simulink model "Thandra_Rushika_prelab5"  (R2022a)
settings: Solver=VariableStepAuto  StartTime=0.0  StopTime=1  RelTol=1e-3
libraries: commanapbnd3 x2
settings Model: Creator=rishika  LastModifiedBy=rishika

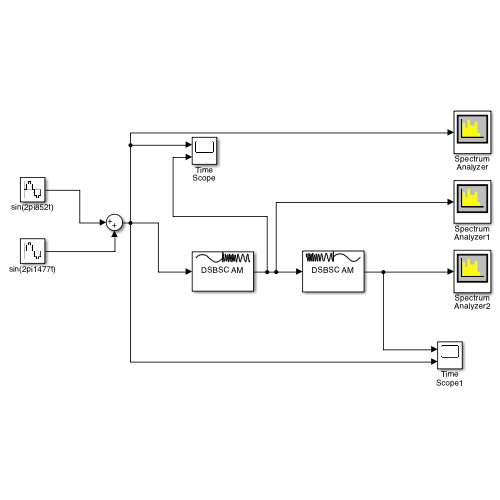
[thumbnail: Simulink's stored preview of the top-level diagram]
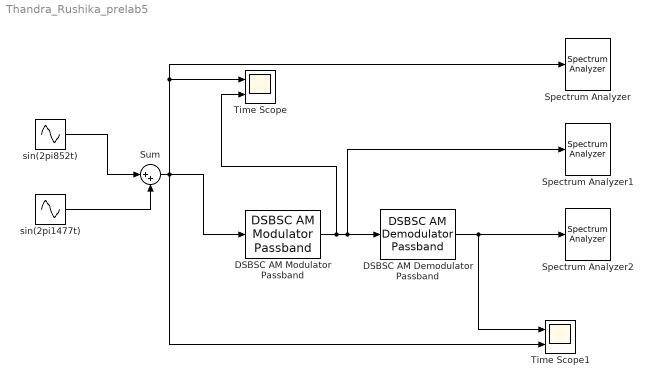
== system Thandra_Rushika_prelab5 ==
  DSBSC AM Demodulator Passband : commanapbnd3/DSBSC AM Demodulator Passband  Fc=8000  Ph=0  method=Butterworth  n=4  cf=5000  Rp=0.1  Rs=50
      settings: SourceProductBaseCode=CM
  DSBSC AM Modulator Passband : commanapbnd3/DSBSC AM Modulator Passband  Fc=8000  Ph=0
      settings: SourceProductBaseCode=CM
  Spectrum Analyzer : SpectrumAnalyzer
  Spectrum Analyzer1 : SpectrumAnalyzer
  Spectrum Analyzer2 : SpectrumAnalyzer
  Sum : Sum  Inputs=|++
  Time Scope : Scope  NumInputPorts=2
  Time Scope1 : Scope  NumInputPorts=2
  sin(2pi1477t) : Sin  Frequency=2*pi*1477  Phase=0.00001  SampleTime=0.00001
  sin(2pi852t) : Sin  Frequency=2*pi*852  SampleTime=0.00001
  wires:
  DSBSC AM Demodulator Passband/1 -> Time Scope1/1, Spectrum Analyzer2/1
  sin(2pi1477t)/1 -> Sum/2
  sin(2pi852t)/1 -> Sum/1
  Sum/1 -> DSBSC AM Modulator Passband/1, Time Scope1/2, Time Scope/1, Spectrum Analyzer/1
  DSBSC AM Modulator Passband/1 -> Time Scope/2, DSBSC AM Demodulator Passband/1, Spectrum Analyzer1/1
